simulink model "model"  (R2020b)
settings: Solver=VariableStepAuto  StartTime=0.0  StopTime=10.0  RelTol=1e-3
settings Model: Creator=SAGAR  LastModifiedBy=SAGAR

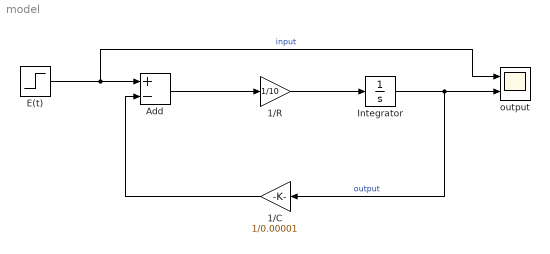
== system model ==
  1/C : Gain  Gain=1/0.00001
  1/R : Gain  Gain=1/10
  Add : Sum  Inputs=+-
  E(t) : Step  After=3  SampleTime=0
  Integrator : Integrator
  output : Scope  NumInputPorts=2
  wires:
  1/R/1 -> Integrator/1
  Add/1 -> 1/R/1
  E(t)/1 -> output/1, Add/1  "input"
  1/C/1 -> Add/2
  Integrator/1 -> output/2, 1/C/1  "output"
